simulink model "tutorial"  (Simulink 5.0)
settings: Solver=ode45  StartTime=0.0  StopTime=10.0  RelTol=1e-3
libraries: cgeqlib x6
settings Model: Creator=CAGE  LastModifiedBy=rlang  BlockReductionOpt=off  BooleanDataType=off

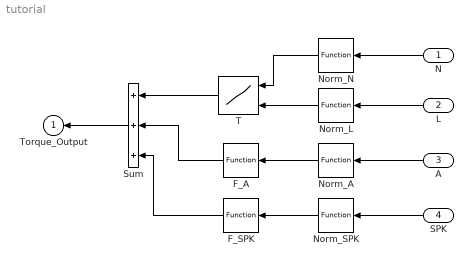
== system tutorial ==
  N : Inport  Orientation=left
      settings: OpenFcn=web(['file:///', which('block_ref.htm')]);
  L : Inport  Orientation=left  Port=2
      settings: OpenFcn=web(['file:///', which('block_ref.htm')]);
  A : Inport  Orientation=left  Port=3
      settings: OpenFcn=web(['file:///', which('block_ref.htm')]);
  SPK : Inport  Orientation=left  Port=4
      settings: OpenFcn=web(['file:///', which('block_ref.htm')]);
  F_A : cgeqlib/Function  Orientation=left
  F_SPK : cgeqlib/Function  Orientation=left
  Norm_A : cgeqlib/Function  Orientation=left
  Norm_L : cgeqlib/Function  Orientation=left
  Norm_N : cgeqlib/Function  Orientation=left
  Norm_SPK : cgeqlib/Function  Orientation=left
  Sum : Sum  Orientation=left  Inputs=+++  SaturateOnIntegerOverflow=on  InputSameDT=on
  T : Lookup2D  Tag=lookuptwo  Orientation=left  RowIndex=[1:3]  ColumnIndex=[1:3]  OutputValues=[4 5 6;16 19 20;10 18 23]  SaturateOnIntegerOverflow=on
  Torque_Output : Outport  Orientation=left
      settings: OpenFcn=callbacks(cgfeaturenode,'i_SLUpdate',[],[],0);
  wires:
  Sum/1 -> Torque_Output/1
  F_A/1 -> Sum/2
  F_SPK/1 -> Sum/3
  T/1 -> Sum/1
  Norm_L/1 -> T/2
  Norm_N/1 -> T/1
  N/1 -> Norm_N/1
  A/1 -> Norm_A/1
  Norm_A/1 -> F_A/1
  Norm_SPK/1 -> F_SPK/1
  L/1 -> Norm_L/1
  SPK/1 -> Norm_SPK/1
